simulink model "PS2_P2_sim"  (R2017a)
settings: Solver=FixedStepAuto  StartTime=0  StopTime=1  FixedStep=.001  RelTol=1e-3
values from neighbouring files (symbols this model uses):
  B = 0.13    [HW2_P1_Mat.m]
  J = 0.01    [HW2_P1_Mat.m]
  K = 52    [HW2_P1_Mat.m]
  theta_0 = 0.175    [HW2_P1_Mat.m]
settings Model: Creator=Shaun  LastModifiedBy=Shaun

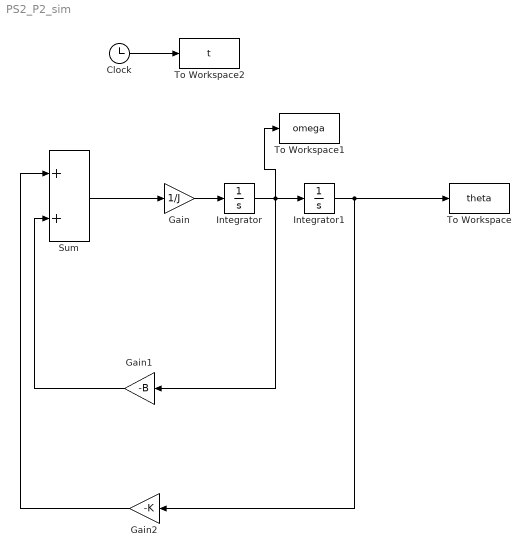
== system PS2_P2_sim ==
  Clock : Clock
      settings: Decimation=5
  Gain : Gain  Gain=1/J
  Gain1 : Gain  Gain=-B
  Gain2 : Gain  Gain=-K
  Integrator : Integrator
  Integrator1 : Integrator  InitialCondition=theta_0
  Sum : Sum
  To Workspace : ToWorkspace  VariableName=theta  SampleTime=-1
  To Workspace1 : ToWorkspace  VariableName=omega  SampleTime=-1
  To Workspace2 : ToWorkspace  VariableName=t  SampleTime=-1
  wires:
  Sum/1 -> Gain/1
  Gain/1 -> Integrator/1
  Integrator/1 -> To Workspace1/1, Gain1/1, Integrator1/1
  Gain1/1 -> Sum/2
  Gain2/1 -> Sum/1
  Integrator1/1 -> To Workspace/1, Gain2/1
  Clock/1 -> To Workspace2/1
